simulink model "camera_test_model_left"  (R2013a)
settings: Solver=ode3  StartTime=0.0  StopTime=T  FixedStep=t_samples  RelTol=1e-3
values from neighbouring files (symbols this model uses):
  t_samples = 0.1    [wide_trajectory.mat]
libraries: vrlib x3, visionsinks x1
settings Model: Creator=HP  LastModifiedBy=HP

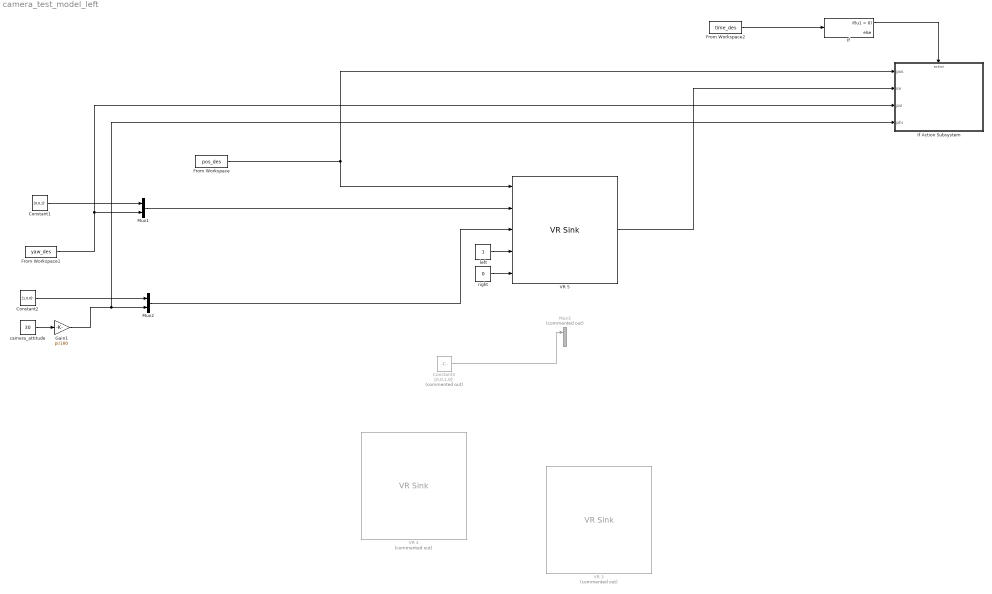
== system camera_test_model_left ==
  Constant1 : Constant  Value=[0,0,1]'
  Constant2 : Constant  Value=[1,0,0]'
  Constant3 : Constant  Commented=on  Value=[0,0,1,0]'
  From Workspace : FromWorkspace  VariableName=pos_des  SampleTime=0
  From Workspace1 : FromWorkspace  VariableName=yaw_des  SampleTime=0
  From Workspace2 : FromWorkspace  VariableName=time_des  SampleTime=0
  Gain1 : Gain  Gain=pi/180
  If : If  SampleTime=t_samples
  If Action Subsystem : Subsystem  TreatAsAtomicUnit=on
  Mux1 : Mux  Inputs=2
  Mux2 : Mux  Inputs=2
  Mux3 : Mux  Commented=on  Inputs=2
  VR 3 : vrlib/VR Sink  Commented=on  InstantiateOnLoad=on  SampleTime=t_samples  ViewEnable=on  RemoteChange=off  RemoteView=off  FieldsWritten=TopView.set_bind.1.1.1.logical#TopView.fieldOfView.1.1.1.double#Drone.translation.3.1.1.double#RotationZ.rotation.4.1.1.double#RotationX.rotation.4.1.1.double#left_cam.set_bind.1.1.1.logical#right_cam.set_bind.1.1.1.logical  WorldFileName=texture\LearningSceneBlue.wrl  AutoView=off  VideoDimensions=[480 640]  AllowVariableSize=off  FigureProperties="{'Position', 'Name', 'Viewpoint', 'CameraBound', 'CameraDirection', 'CameraPosition', 'CameraUpVector', 'ZoomFactor', 'Antialiasing', 'Headlight', 'Lighting', 'NavPanel', 'StatusBar', 'ToolBar', 'Textures', 'Transparency', 'Triad', 'Wireframe', 'NavZones', 'NavMode', 'NavSpeed', 'CaptureFileFormat', 'CaptureFileName', 'Record2DCompressMethod', 'Record2DCompressQuality', 'Record2D', 'Record2DFileName', 'Record2DFPS'; [3.0000000000000000e+01   6.0000000000000000e+01   6.4000000000000000e+02   4.8000000000000000e+02], '', 'right_cam', 'on', [0.0000000000000000e+00   0.0000000000000000e+00  -1.0000000000000000e+00], [0.0000000000000000e+00   0.0000000000000000e+00   0.0000000000000000e+00], [0.0000000000000000e+00   1.0000000000000000e+00   0.0000000000000000e+00], [1.0000000000000000e+00], 'on', 'on', 'on', 'none', 'off', 'off', 'on', 'on', 'none', 'off', 'off', 'examine', 'normal', 'tif', '%f_anim_%n.tif', 'auto', [7.5000000000000000e+01], 'off', '***video***', [1.5000000000000000e+01]}"
  VR 4 : vrlib/VR Sink  Commented=on  InstantiateOnLoad=on  SampleTime=t_samples  ViewEnable=on  RemoteChange=off  RemoteView=off  FieldsWritten=Drone.translation.3.1.1.double#RotationZ.rotation.4.1.1.double#RotationX.rotation.4.1.1.double#left_cam.set_bind.1.1.1.logical#right_cam.set_bind.1.1.1.logical  WorldFileName=texture\LearningScene4Wpts.wrl  AutoView=off  VideoDimensions=[480 640]  AllowVariableSize=off  FigureProperties="{'Position', 'Name', 'Viewpoint', 'CameraBound', 'CameraDirection', 'CameraPosition', 'CameraUpVector', 'ZoomFactor', 'Antialiasing', 'Headlight', 'Lighting', 'NavPanel', 'StatusBar', 'ToolBar', 'Textures', 'Transparency', 'Triad', 'Wireframe', 'NavZones', 'NavMode', 'NavSpeed', 'CaptureFileFormat', 'CaptureFileName', 'Record2DCompressMethod', 'Record2DCompressQuality', 'Record2D', 'Record2DFileName', 'Record2DFPS'; [3.0000000000000000e+01   6.0000000000000000e+01   6.4000000000000000e+02   4.8000000000000000e+02], '', 'right_cam', 'on', [0.0000000000000000e+00   0.0000000000000000e+00  -1.0000000000000000e+00], [0.0000000000000000e+00   0.0000000000000000e+00   0.0000000000000000e+00], [0.0000000000000000e+00   1.0000000000000000e+00   0.0000000000000000e+00], [1.0000000000000000e+00], 'on', 'on', 'on', 'none', 'off', 'off', 'on', 'on', 'none', 'off', 'off', 'examine', 'normal', 'tif', '%f_anim_%n.tif', 'auto', [7.5000000000000000e+01], 'off', '***video***', [1.5000000000000000e+01]}"
  "VR 5 " : vrlib/VR Sink  InstantiateOnLoad=on  SampleTime=t_samples  ViewEnable=on  RemoteChange=off  RemoteView=off  FieldsWritten=Drone.translation.3.1.1.double#RotationZ.rotation.4.1.1.double#RotationX.rotation.4.1.1.double#left_cam.set_bind.1.1.1.logical#right_cam.set_bind.1.1.1.logical  WorldFileName=LearningSceneWide.wrl  AutoView=off  VideoDimensions=[480 640]  AllowVariableSize=off  FigureProperties="{'Position', 'Name', 'Viewpoint', 'CameraBound', 'CameraDirection', 'CameraPosition', 'CameraUpVector', 'ZoomFactor', 'Antialiasing', 'Headlight', 'Lighting', 'NavPanel', 'StatusBar', 'ToolBar', 'Textures', 'Transparency', 'Triad', 'Wireframe', 'NavZones', 'NavMode', 'NavSpeed', 'CaptureFileFormat', 'CaptureFileName', 'Record2DCompressMethod', 'Record2DCompressQuality', 'Record2D', 'Record2DFileName', 'Record2DFPS'; [3.0000000000000000e+01   6.0000000000000000e+01   6.4000000000000000e+02   4.8000000000000000e+02], '', 'left_cam', 'on', [0.0000000000000000e+00   0.0000000000000000e+00  -1.0000000000000000e+00], [0.0000000000000000e+00   0.0000000000000000e+00   0.0000000000000000e+00], [0.0000000000000000e+00   1.0000000000000000e+00   0.0000000000000000e+00], [1.0000000000000000e+00], 'on', 'on', 'on', 'none', 'off', 'off', 'on', 'on', 'none', 'off', 'off', 'examine', 'normal', 'tif', '%f_anim_%n.tif', 'auto', [7.5000000000000000e+01], 'off', '***video***', [1.5000000000000000e+01]}"
  camera_attitude : Constant  Value=30
  left : Constant  SampleTime=-1
  "right " : Constant  Value=0
  wires:
  left/1 -> "VR 5 "/4
  "right "/1 -> "VR 5 "/5
  Constant1/1 -> Mux1/1
  From Workspace1/1 -> If Action Subsystem/3(psi), Mux1/2
  Constant2/1 -> Mux2/1
  camera_attitude/1 -> Gain1/1
  Gain1/1 -> If Action Subsystem/4(phi), Mux2/2
  Constant3/1 -> Mux3/1
  Mux1/1 -> "VR 5 "/2
  Mux2/1 -> "VR 5 "/3
  From Workspace/1 -> If Action Subsystem/1(pos), "VR 5 "/1
  "VR 5 "/1 -> If Action Subsystem/2(im)
  ? -> ?
  If/1 -> If Action Subsystem/Action
  From Workspace2/1 -> If/1

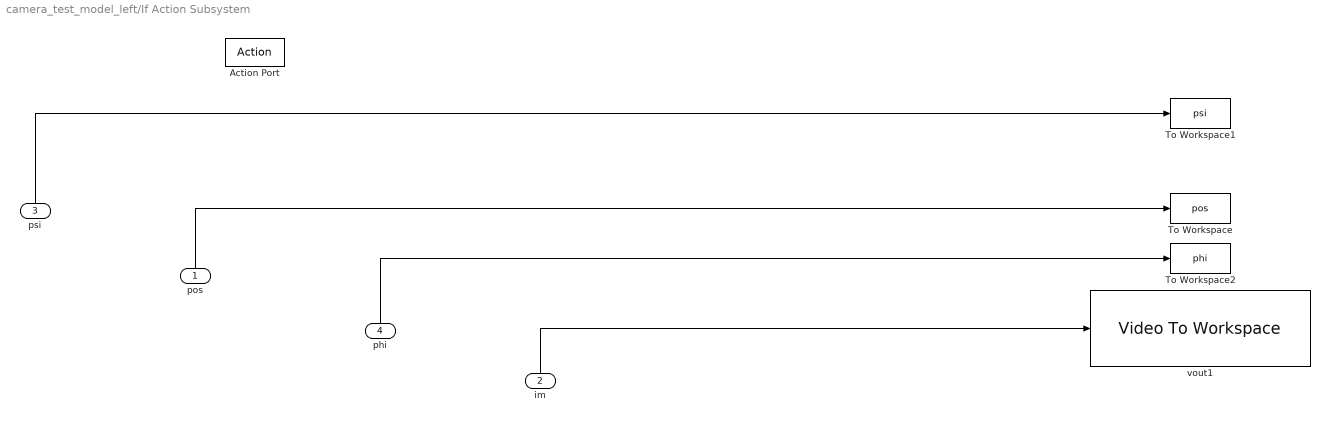
== system camera_test_model_left/If Action Subsystem ==
  pos : Inport
  im : Inport  Port=2
  psi : Inport  Port=3
  phi : Inport  Port=4
  Action Port : ActionPort  ActionType=then
  To Workspace : ToWorkspace  VariableName=pos  SampleTime=t_samples  SaveFormat=Structure
  To Workspace1 : ToWorkspace  VariableName=psi  SampleTime=t_samples  SaveFormat=Structure
  To Workspace2 : ToWorkspace  VariableName=phi  SampleTime=t_samples  SaveFormat=Structure
  vout1 : visionsinks/Video To Workspace  VariableName=vout_left  NumInputs=1  DataLimit=inf  DecimationFactor=1  LogFi=off  InPortLabels=R|G|B
  wires:
  psi/1 -> To Workspace1/1
  pos/1 -> To Workspace/1
  phi/1 -> To Workspace2/1
  im/1 -> vout1/1
